simulink model "impedanceControl"  (R2016b)
settings: Solver=FixedStepDiscrete  StartTime=0.0  StopTime=CONFIG.SIMULATION_TIME  FixedStep=Ts  RelTol=1e-3  EnableMultiTasking=on
InitFcn:
  | cd(fileparts(which(bdroot)));
  | init_impedanceControl;
values from neighbouring files (symbols this model uses):
  FRIC_COMP = 1    [init_impedanceControl.m]
  GRAV_COMP = 1    [init_impedanceControl.m]
  MOVING = 0    [init_impedanceControl.m]
undefined symbols (not defined in the file or in its folder): AMPLS, FREQS, Kd, Kp, ROBOT_DOF
libraries: WBToolboxLibrary x12
settings Model: Creator=daniele  LastModifiedBy=marie
settings DataIOCC: LimitDataPoints=on  SaveFormat=Array  SignalLoggingSaveFormat=ModelDataLogs
settings OptimizationCC: LifeSpan=inf
settings DebuggingCC: SolverPrmCheckMsg=warning  MultiTaskDSMMsg=warning  MultiTaskCondExecSysMsg=none  AllowSymbolicDim=off  StrictBusMsg=ErrorOnBusTreatedAsVector  SFUnexpectedBacktrackingDiag=warning  SFNoUnconditionalDefaultTransitionDiag=warning  SFExecutionAtInitializationDiag=none
settings HardwareCC: ProdBitPerPointer=32  ProdBitPerSizeT=32  ProdBitPerPtrDiffT=32  ProdLargestAtomicFloat=None  ProdIntDivRoundTo=Undefined  ProdEndianess=Unspecified  ProdWordSize=32  ProdHWDeviceType=32-bit Generic
settings ModelReferenceCC: PropagateSignalLabelsOutOfModel=off
settings GRTTargetCC: TargetLangStandard=C89/C90 (ANSI)  GeneratePreprocessorConditionals=Disable all
settings ConfigComp: CovMetricSettings=dw  CovHtmlReporting=on  CovSaveCumulativeToWorkspaceVar=on  CovSaveSingleToWorkspaceVar=on  CovExternalEMLEnable=off

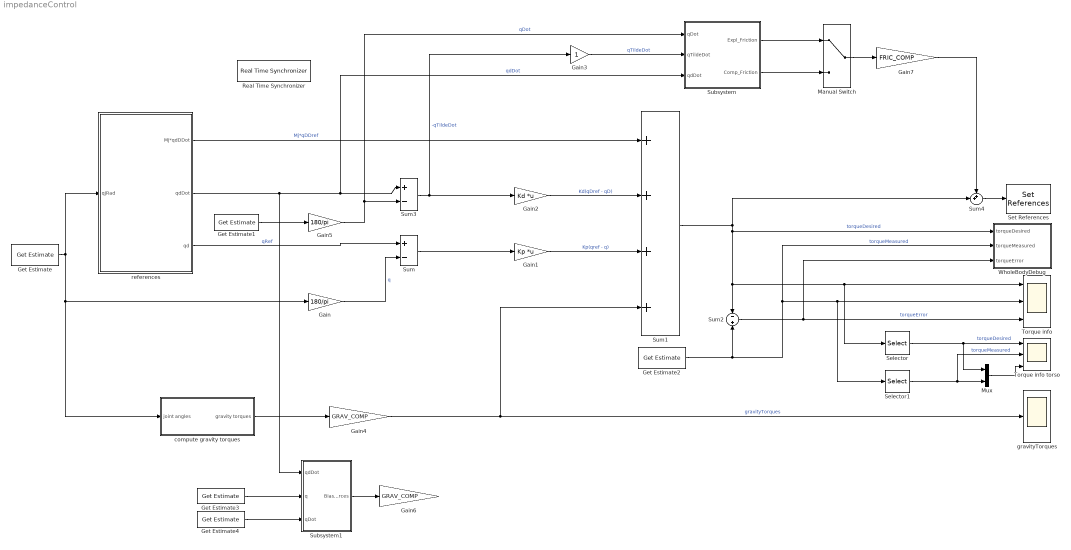
== system impedanceControl ==
  Gain : Gain  Gain=180/pi
  Gain1 : Gain  Gain=Kp  Multiplication=Matrix(K*u)
  Gain2 : Gain  Gain=Kd  Multiplication=Matrix(K*u)
  Gain3 : Gain
  Gain4 : Gain  Gain=GRAV_COMP
  Gain5 : Gain  Gain=180/pi
  Gain6 : Gain  Gain=GRAV_COMP
  Gain7 : Gain  Gain=FRIC_COMP
  Get Estimate : WBToolboxLibrary/wholeBodyStates/Get Estimate  estimateType=Joints Position  robotName=WBT_robotName  localName=WBT_modelName  wbiFile=WBT_wbiFilename  wbiList=WBT_wbiList
  Get Estimate1 : WBToolboxLibrary/wholeBodyStates/Get Estimate  estimateType=Joints Velocity  robotName=WBT_robotName  localName=WBT_modelName  wbiFile=WBT_wbiFilename  wbiList=WBT_wbiList
  Get Estimate2 : WBToolboxLibrary/wholeBodyStates/Get Estimate  estimateType=Joints Torque  robotName=WBT_robotName  localName=WBT_modelName  wbiFile=WBT_wbiFilename  wbiList=WBT_wbiList
  Get Estimate3 : WBToolboxLibrary/wholeBodyStates/Get Estimate  estimateType=Joints Position  robotName=WBT_robotName  localName=WBT_modelName  wbiFile=WBT_wbiFilename  wbiList=WBT_wbiList
  Get Estimate4 : WBToolboxLibrary/wholeBodyStates/Get Estimate  estimateType=Joints Velocity  robotName=WBT_robotName  localName=WBT_modelName  wbiFile=WBT_wbiFilename  wbiList=WBT_wbiList
  Manual Switch : ManualSwitch
  Mux : Mux  Inputs=2
  Real Time Synchronizer : WBToolboxLibrary/Utilities/Real Time Synchronizer  period=0.01
  Selector : Selector  InputPortWidth=ROBOT_DOF  IndexOptions=Index vector (dialog)  Indices=[1 2 3]  OutputSizes=1
  Selector1 : Selector  InputPortWidth=ROBOT_DOF  IndexOptions=Index vector (dialog)  Indices=[1 2 3]  OutputSizes=1
  Set References : WBToolboxLibrary/wholeBodyActuators/Set References  controlType=Torque  fullOrSubControl=Full  controlledJoints=''  robotName=WBT_robotName  localName=WBT_modelName  wbiFile=WBT_wbiFilename  wbiList=WBT_wbiList
  Subsystem : Subsystem
  Subsystem1 : Subsystem
  Sum : Sum  Inputs=+-
  Sum1 : Sum  Inputs=++++
  Sum2 : Sum  Inputs=-|+
  Sum3 : Sum  Inputs=+-
  Sum4 : Sum  Inputs=++|
  Torque info : Scope  NumInputPorts=3
  Torque info torso : Scope  NumInputPorts=3
  WholeBodyDebug : Subsystem
  compute gravity torques : Subsystem
  gravityTorques : Scope
  references : Subsystem
  wires:
  Gain/1 -> Sum/2  "q"
  Sum/1 -> Gain1/1
  Gain1/1 -> Sum1/3  "Kp(qref - q)"
  Gain2/1 -> Sum1/2  "Kd(qDref - qD)"
  Get Estimate/1 -> compute gravity torques/1(joint angles), Gain/1, references/1(qjRad)
  Get Estimate2/1 -> WholeBodyDebug/2(torqueMeasured), Selector1/1, Torque info/2, Sum2/2  "torqueMeasured"
  Sum2/1 -> WholeBodyDebug/3(torqueError), Torque info/3  "torqueError"
  references/3(" qd") -> Sum/1  "qRef"
  Gain5/1 -> Subsystem/1(qDot), Sum3/2  "qDot"
  Sum3/1 -> Gain2/1, Gain3/1  "-qTildeDot"
  references/2(qdDot) -> Subsystem/3(qdDot), Sum3/1, Subsystem1/1(qdDot)  "qdDot"
  references/1(Mj*qdDDot) -> Sum1/1  "Mj*qDDref"
  Gain4/1 -> Sum1/4, gravityTorques/1  "gravityTorques"
  Get Estimate1/1 -> Gain5/1
  compute gravity torques/1(gravity torques) -> Gain4/1
  Sum1/1 -> WholeBodyDebug/1(torqueDesired), Sum2/1, Selector/1, Torque info/1, Sum4/2  "torqueDesired"
  Selector/1 -> Torque info torso/1, Mux/1  "torqueDesired"
  Selector1/1 -> Torque info torso/2, Mux/2  "torqueMeasured"
  Mux/1 -> Torque info torso/3
  Sum4/1 -> Set References/1
  Gain3/1 -> Subsystem/2(qTildeDot)  "qTildeDot"
  Manual Switch/1 -> Gain7/1
  Subsystem/1("Expl_Friction ") -> Manual Switch/1
  Subsystem/2(Comp_Friction) -> Manual Switch/2
  Get Estimate3/1 -> Subsystem1/2(q)
  Get Estimate4/1 -> Subsystem1/3(qDot)
  Subsystem1/1(Bias Forces) -> Gain6/1
  Gain7/1 -> Sum4/1

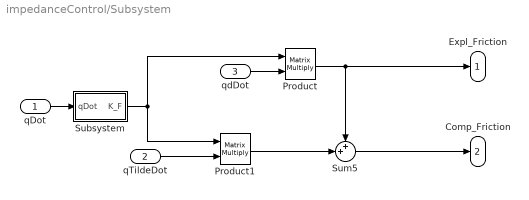
== system impedanceControl/Subsystem ==
  qDot : Inport
  qTildeDot : Inport  Port=2
  qdDot : Inport  Port=3
  Product : Product  Multiplication=Matrix(*)
  Product1 : Product  Multiplication=Matrix(*)
  Subsystem : Subsystem
  Sum5 : Sum  Inputs=++|
  "Expl_Friction " : Outport
  Comp_Friction : Outport  Port=2
  wires:
  qdDot/1 -> Product/2
  Product/1 -> "Expl_Friction "/1, Sum5/1
  Sum5/1 -> Comp_Friction/1
  Product1/1 -> Sum5/2
  qTildeDot/1 -> Product1/2
  Subsystem/1(K_F) -> Product1/1, Product/1
  qDot/1 -> Subsystem/1(qDot)

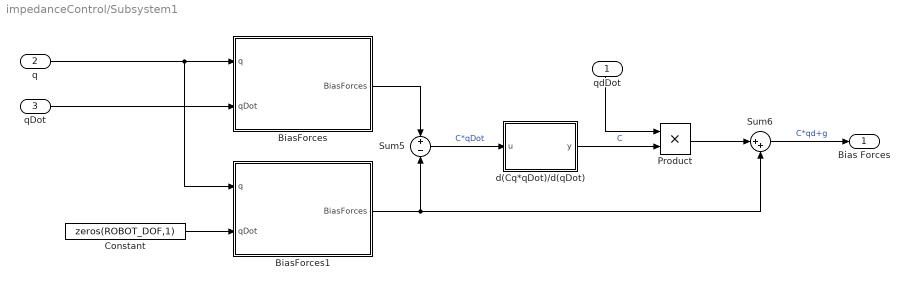
== system impedanceControl/Subsystem1 ==
  qdDot : Inport  PortDimensions=ROBOT_DOF
  q : Inport  Port=2
  qDot : Inport  Port=3
  " d(Cq*qDot)/d(qDot)" : MATLAB Function  TreatAsAtomicUnit=on
  BiasForces : Subsystem
  BiasForces1 : Subsystem
  Constant : Constant  Value=zeros(ROBOT_DOF,1)
  Product : Product
  Sum5 : Sum  Inputs=+|-
  Sum6 : Sum  Inputs=|++
  Bias Forces : Outport
  wires:
  " d(Cq*qDot)/d(qDot)"/1(y) -> Product/2  "C"
  Sum5/1 -> " d(Cq*qDot)/d(qDot)"/1(u)  "C*qDot"
  q/1 -> BiasForces1/1(q), BiasForces/1(q)
  qDot/1 -> BiasForces/2(qDot)
  Constant/1 -> BiasForces1/2(qDot)
  BiasForces/1(BiasForces) -> Sum5/1
  Product/1 -> Sum6/1
  BiasForces1/1(BiasForces) -> Sum6/2, Sum5/2
  qdDot/1 -> Product/1
  Sum6/1 -> Bias Forces/1  "C*qd+g"

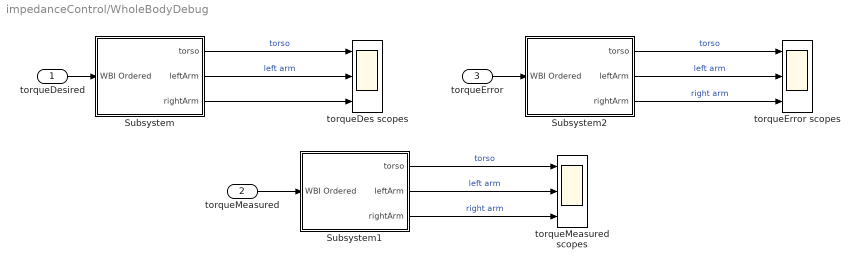
== system impedanceControl/WholeBodyDebug ==
  torqueDesired : Inport
  torqueMeasured : Inport  Port=2
  torqueError : Inport  Port=3
  Subsystem : Subsystem
  Subsystem1 : Subsystem
  Subsystem2 : Subsystem
  torqueDes scopes : Scope  NumInputPorts=3
  "torqueError scopes  " : Scope  NumInputPorts=3
  "torqueMeasured scopes  " : Scope  NumInputPorts=3
  wires:
  torqueMeasured/1 -> Subsystem1/1(WBI Ordered)
  torqueError/1 -> Subsystem2/1(WBI Ordered)
  torqueDesired/1 -> Subsystem/1(WBI Ordered)
  Subsystem/1(torso) -> torqueDes scopes/1  "torso"
  Subsystem/2(leftArm) -> torqueDes scopes/2  "left arm"
  Subsystem1/1(torso) -> "torqueMeasured scopes  "/1  "torso"
  Subsystem1/2(leftArm) -> "torqueMeasured scopes  "/2  "left arm"
  Subsystem1/3(rightArm) -> "torqueMeasured scopes  "/3  "right arm"
  Subsystem2/1(torso) -> "torqueError scopes  "/1  "torso"
  Subsystem2/2(leftArm) -> "torqueError scopes  "/2  "left arm"
  Subsystem2/3(rightArm) -> "torqueError scopes  "/3  "right arm"
  Subsystem/3(rightArm) -> torqueDes scopes/3

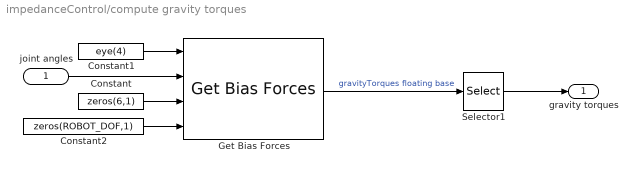
== system impedanceControl/compute gravity torques ==
  joint angles : Inport
  Constant : Constant  Value=zeros(6,1)
  Constant1 : Constant  Value=eye(4)
  Constant2 : Constant  Value=zeros(ROBOT_DOF,1)
  Get Bias Forces : WBToolboxLibrary/wholeBodyModel/Dynamics/Get Bias Forces  robotName=WBT_robotName  localName=WBT_modelName  wbiFile=WBT_wbiFilename  wbiList=WBT_wbiList  explicitGravity=off
  Selector1 : Selector  InputPortWidth=ROBOT_DOF+6  IndexOptions=Index vector (dialog)  Indices=[7:ROBOT_DOF+6]  OutputSizes=1
  gravity torques : Outport
  wires:
  Selector1/1 -> gravity torques/1
  Constant1/1 -> Get Bias Forces/1
  Constant2/1 -> Get Bias Forces/4
  joint angles/1 -> Get Bias Forces/2
  Constant/1 -> Get Bias Forces/3
  Get Bias Forces/1 -> Selector1/1  "gravityTorques floating base"

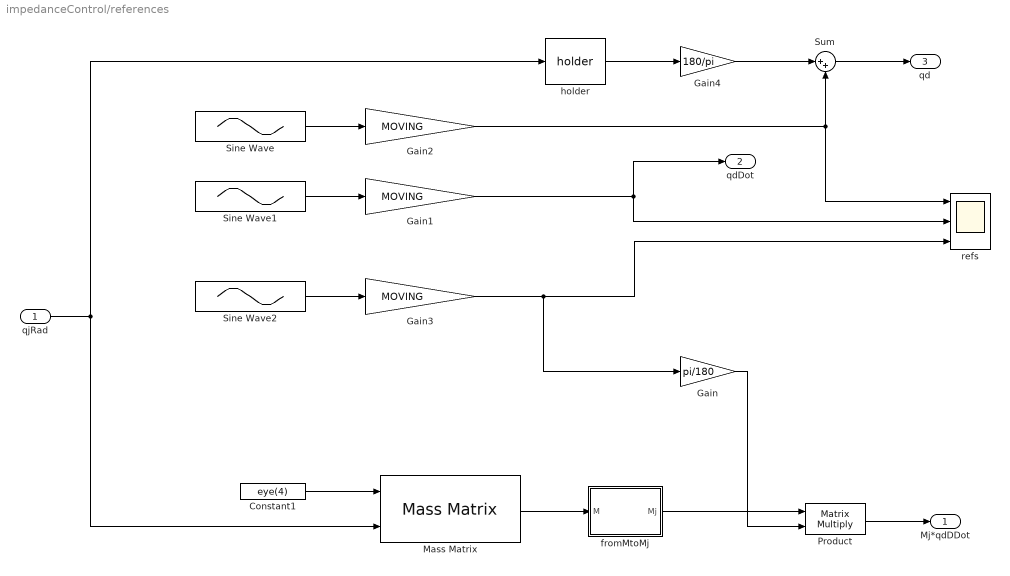
== system impedanceControl/references ==
  qjRad : Inport
  Constant1 : Constant  Value=eye(4)
  Gain : Gain  Gain=pi/180
  Gain1 : Gain  Gain=MOVING
  Gain2 : Gain  Gain=MOVING
  Gain3 : Gain  Gain=MOVING
  Gain4 : Gain  Gain=180/pi
  Mass Matrix : WBToolboxLibrary/wholeBodyModel/Dynamics/Mass Matrix  robotName=WBT_robotName  localName=WBT_modelName  wbiFile=WBT_wbiFilename  wbiList=WBT_wbiList
  Product : Product  Multiplication=Matrix(*)
  Sine Wave : Sin  Amplitude=AMPLS  Frequency=FREQS*2*pi  SampleTime=0
  Sine Wave1 : Sin  Amplitude=AMPLS.*FREQS*2*pi  Frequency=FREQS*2*pi  Phase=pi/2  SampleTime=0
  Sine Wave2 : Sin  Amplitude=-AMPLS.*(FREQS*2*pi).^2  Frequency=FREQS*2*pi  SampleTime=0
  Sum : Sum  Inputs=|++
  fromMtoMj : MATLAB Function  TreatAsAtomicUnit=on
  "holder " : WBToolboxLibrary/Utilities/holder 
  refs : Scope  NumInputPorts=3
  Mj*qdDDot : Outport
  qdDot : Outport  Port=2
  " qd" : Outport  Port=3
  wires:
  Sine Wave/1 -> Gain2/1
  Gain2/1 -> Sum/2, refs/1
  Sine Wave1/1 -> Gain1/1
  Gain1/1 -> refs/2, qdDot/1
  Sine Wave2/1 -> Gain3/1
  Product/1 -> Mj*qdDDot/1
  Mass Matrix/1 -> fromMtoMj/1(M)
  fromMtoMj/1(Mj) -> Product/1
  Gain3/1 -> refs/3, Gain/1
  Gain/1 -> Product/2
  qjRad/1 -> "holder "/1, Mass Matrix/2
  Sum/1 -> " qd"/1
  "holder "/1 -> Gain4/1
  Gain4/1 -> Sum/1
  Constant1/1 -> Mass Matrix/1

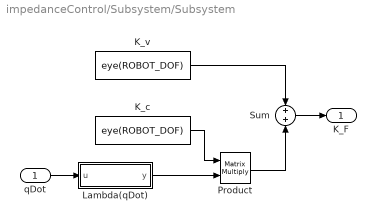
== system impedanceControl/Subsystem/Subsystem ==
  qDot : Inport
  K_c : Constant  Value=eye(ROBOT_DOF)
  K_v : Constant  Value=eye(ROBOT_DOF)
  Lambda(qDot) : MATLAB Function  TreatAsAtomicUnit=on
  Product : Product  Multiplication=Matrix(*)
  Sum : Sum  Inputs=+|+
  K_F : Outport
  wires:
  K_v/1 -> Sum/1
  Sum/1 -> K_F/1
  qDot/1 -> Lambda(qDot)/1(u)
  Product/1 -> Sum/2
  K_c/1 -> Product/1
  Lambda(qDot)/1(y) -> Product/2

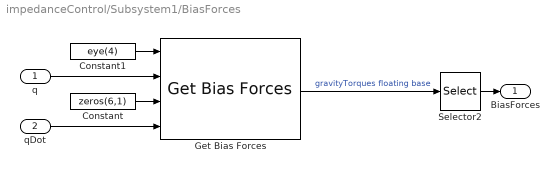
== system impedanceControl/Subsystem1/BiasForces ==
  q : Inport
  qDot : Inport  Port=2
  Constant : Constant  Value=zeros(6,1)
  Constant1 : Constant  Value=eye(4)
  Get Bias Forces : WBToolboxLibrary/wholeBodyModel/Dynamics/Get Bias Forces  robotName=WBT_robotName  localName=WBT_modelName  wbiFile=WBT_wbiFilename  wbiList=WBT_wbiList  explicitGravity=off
  Selector2 : Selector  InputPortWidth=ROBOT_DOF+6  IndexOptions=Index vector (dialog)  Indices=[7:ROBOT_DOF+6]  OutputSizes=1
  BiasForces : Outport
  wires:
  Constant/1 -> Get Bias Forces/3
  q/1 -> Get Bias Forces/2
  Selector2/1 -> BiasForces/1
  qDot/1 -> Get Bias Forces/4
  Constant1/1 -> Get Bias Forces/1
  Get Bias Forces/1 -> Selector2/1  "gravityTorques floating base"

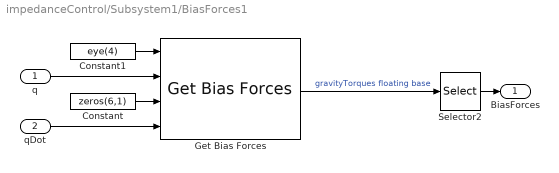
== system impedanceControl/Subsystem1/BiasForces1 ==
  q : Inport
  qDot : Inport  Port=2
  Constant : Constant  Value=zeros(6,1)
  Constant1 : Constant  Value=eye(4)
  Get Bias Forces : WBToolboxLibrary/wholeBodyModel/Dynamics/Get Bias Forces  robotName=WBT_robotName  localName=WBT_modelName  wbiFile=WBT_wbiFilename  wbiList=WBT_wbiList  explicitGravity=off
  Selector2 : Selector  InputPortWidth=ROBOT_DOF+6  IndexOptions=Index vector (dialog)  Indices=[7:ROBOT_DOF+6]  OutputSizes=1
  BiasForces : Outport
  wires:
  Constant/1 -> Get Bias Forces/3
  q/1 -> Get Bias Forces/2
  Selector2/1 -> BiasForces/1
  qDot/1 -> Get Bias Forces/4
  Constant1/1 -> Get Bias Forces/1
  Get Bias Forces/1 -> Selector2/1  "gravityTorques floating base"

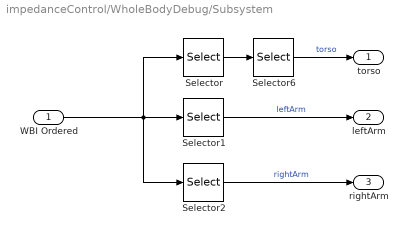
== system impedanceControl/WholeBodyDebug/Subsystem ==
  WBI Ordered : Inport
  Selector : Selector  InputPortWidth=ROBOT_DOF  IndexOptions=Index vector (dialog)  Indices=[1:3]  OutputSizes=1
  Selector1 : Selector  InputPortWidth=ROBOT_DOF  IndexOptions=Index vector (dialog)  Indices=[4:7]  OutputSizes=1
  Selector2 : Selector  InputPortWidth=ROBOT_DOF  IndexOptions=Index vector (dialog)  Indices=[8:11]  OutputSizes=1
  Selector6 : Selector  InputPortWidth=3  IndexOptions=Index vector (dialog)  Indices=[3 2 1]  OutputSizes=1
  torso : Outport
  leftArm : Outport  Port=2
  rightArm : Outport  Port=3
  wires:
  Selector/1 -> Selector6/1
  Selector1/1 -> leftArm/1  "leftArm"
  Selector6/1 -> torso/1  "torso"
  Selector2/1 -> rightArm/1  "rightArm"
  WBI Ordered/1 -> Selector2/1, Selector1/1, Selector/1

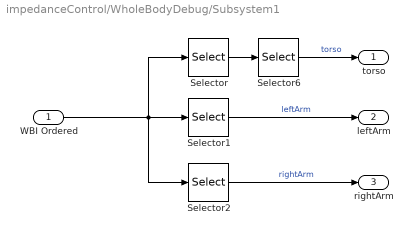
== system impedanceControl/WholeBodyDebug/Subsystem1 ==
  WBI Ordered : Inport
  Selector : Selector  InputPortWidth=ROBOT_DOF  IndexOptions=Index vector (dialog)  Indices=[1:3]  OutputSizes=1
  Selector1 : Selector  InputPortWidth=ROBOT_DOF  IndexOptions=Index vector (dialog)  Indices=[4:7]  OutputSizes=1
  Selector2 : Selector  InputPortWidth=ROBOT_DOF  IndexOptions=Index vector (dialog)  Indices=[8:11]  OutputSizes=1
  Selector6 : Selector  InputPortWidth=3  IndexOptions=Index vector (dialog)  Indices=[3 2 1]  OutputSizes=1
  torso : Outport
  leftArm : Outport  Port=2
  rightArm : Outport  Port=3
  wires:
  Selector/1 -> Selector6/1
  Selector1/1 -> leftArm/1  "leftArm"
  Selector6/1 -> torso/1  "torso"
  Selector2/1 -> rightArm/1  "rightArm"
  WBI Ordered/1 -> Selector2/1, Selector1/1, Selector/1

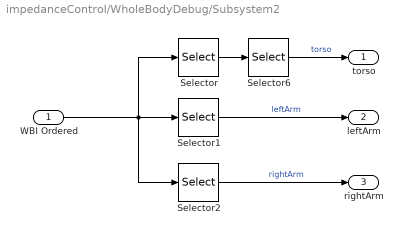
== system impedanceControl/WholeBodyDebug/Subsystem2 ==
  WBI Ordered : Inport
  Selector : Selector  InputPortWidth=ROBOT_DOF  IndexOptions=Index vector (dialog)  Indices=[1:3]  OutputSizes=1
  Selector1 : Selector  InputPortWidth=ROBOT_DOF  IndexOptions=Index vector (dialog)  Indices=[4:7]  OutputSizes=1
  Selector2 : Selector  InputPortWidth=ROBOT_DOF  IndexOptions=Index vector (dialog)  Indices=[8:11]  OutputSizes=1
  Selector6 : Selector  InputPortWidth=3  IndexOptions=Index vector (dialog)  Indices=[3 2 1]  OutputSizes=1
  torso : Outport
  leftArm : Outport  Port=2
  rightArm : Outport  Port=3
  wires:
  Selector/1 -> Selector6/1
  Selector1/1 -> leftArm/1  "leftArm"
  Selector6/1 -> torso/1  "torso"
  Selector2/1 -> rightArm/1  "rightArm"
  WBI Ordered/1 -> Selector2/1, Selector1/1, Selector/1

== matlab function impedanceControl/Subsystem1/ d(Cq*qDot)//d(qDot) ==
  data: u input; y output
function y = fcn(u)

y = u;

== matlab function impedanceControl/references/fromMtoMj ==
  data: M input; Mj output
function Mj = fromMtoMj(M)
%#codegen

Mj = M(7:end,7:end);

== matlab function impedanceControl/Subsystem/Subsystem/Lambda(qDot) ==
  data: u input; y output
function y = fcn(u)

y = diag(1./abs(u));
